simulink model "half_controlled_model"  (R2021b)
settings: Solver=VariableStepAuto  StartTime=0.0  StopTime=2  RelTol=1e-3
undefined symbols (not defined in the file): magnitude
libraries: spsCurrentMeasurementLib x2, spsDiodeLib x2, spsMeanLib x2, spsSeriesRLCBranchLib x2, spsThyristorLib x2, spsVoltageMeasurementLib x2, spsACVoltageSourceLib x1, spsDCMachineLib x1, spsDCVoltageSourceLib x1, spspowerguiLib x1
settings Model: Creator=ardak  LastModifiedBy=ardak

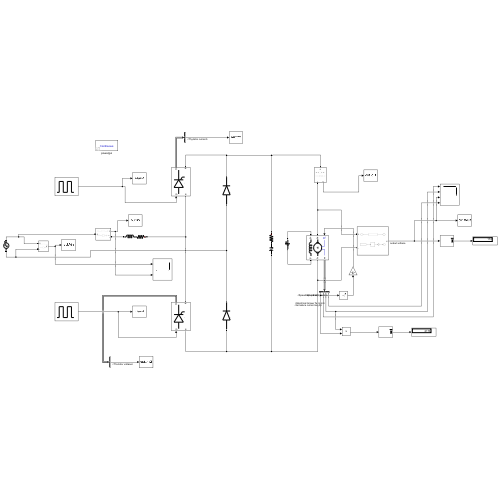
[thumbnail: Simulink's stored preview of the top-level diagram]
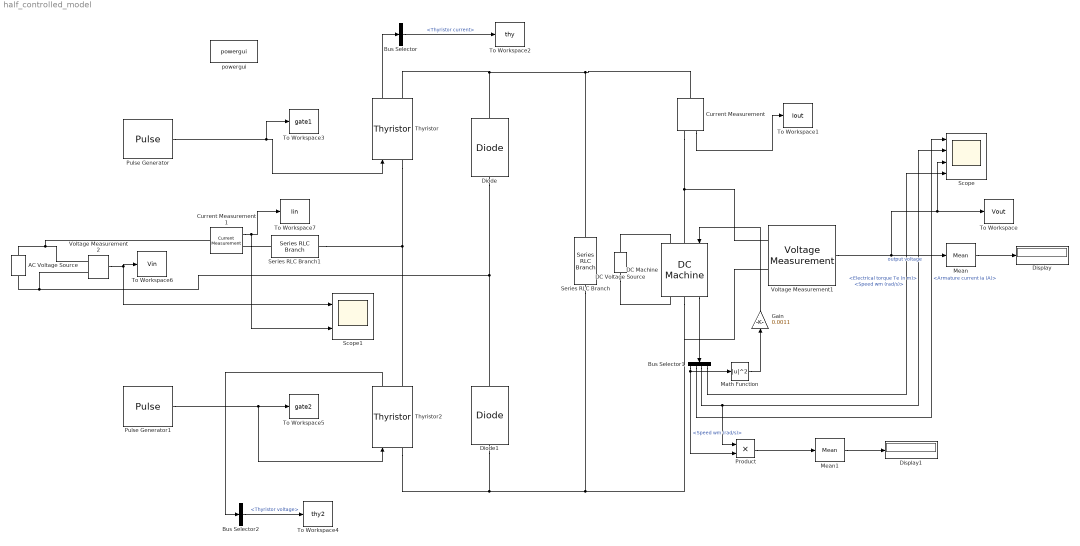
== system half_controlled_model ==
  AC Voltage Source : spsACVoltageSourceLib/AC Voltage Source  Amplitude=230*sqrt(2)  Phase=0  Frequency=50  SampleTime=1e-6  Measurements=None  BusType=swing  Pref=10e3  Qref=0  Qmin=-inf  Qmax=+inf
  Bus Selector : BusSelector  OutputSignals=Thyristor current
  Bus Selector1 : BusSelector  OutputSignals=Speed wm (rad/s),Armature current ia (A),Electrical torque Te (n m),Speed wm (rad/s)
  Bus Selector2 : BusSelector  OutputSignals=Thyristor voltage
  Current Measurement : spsCurrentMeasurementLib/Current Measurement  PhasorSimulation=off  OutputType=Complex  PSBequivalent=0
  Current Measurement1 : spsCurrentMeasurementLib/Current Measurement  PhasorSimulation=off  OutputType=Complex  PSBequivalent=0
  DC Machine : spsDCMachineLib/DC Machine  PresetModel=No  MechanicalLoad=Torque TL  FieldType=Wound  ShowDetailedParameters=on  MeasurementBus=off  RLa="[ 0.8  0.0125]"  RLf="[ 210  23]"  Laf=1.8  MachineConstant=Torque constant (N.m/A)  Ke=1.8  Kt=1.8  J=0.022  Bm=0.002953  Tf=0.5161  w0=1  Ifinit=0.714285714285714  TsPowergui=0  TsBlock=-1
  DC Voltage Source : spsDCVoltageSourceLib/DC Voltage Source  Amplitude=150  Measurements=None
  Diode : spsDiodeLib/Diode  Ron=0  Lon=0  Vf=1.2  IC=0  UseSnubber=0  Rs=inf  Cs=inf  Measurements=off
  Diode1 : spsDiodeLib/Diode  Ron=0  Lon=0  Vf=1.2  IC=0  UseSnubber=0  Rs=inf  Cs=inf  Measurements=off
  Display : Display
  Display1 : Display
  Gain : Gain  Gain=0.0011
  Math Function : Math  Operator=magnitude^2  SaturateOnIntegerOverflow=on
  Mean : spsMeanLib/Mean  Freq=60  Vinit=0  Ts=0
  Mean1 : spsMeanLib/Mean  Freq=60  Vinit=0  Ts=0
  Product : Product
  Pulse Generator : DiscretePulseGenerator  PulseType=Time based  Amplitude=200  Period=0.02  PulseWidth=20  PhaseDelay=0.0035
  Pulse Generator1 : DiscretePulseGenerator  PulseType=Time based  Amplitude=200  Period=0.02  PulseWidth=20  PhaseDelay=0.0135
  Scope : Scope  NumInputPorts=4
  Scope1 : Scope  NumInputPorts=2
  Series RLC Branch : spsSeriesRLCBranchLib/Series RLC Branch  LConnTagsString=__new0  RConnTagsString=__new0  BranchType=RC  Resistance=1  Inductance=1e-3  SetiL0=off  InitialCurrent=0  Capacitance=1360e-6  Setx0=off  InitialVoltage=0  Measurements=None
  Series RLC Branch1 : spsSeriesRLCBranchLib/Series RLC Branch  LConnTagsString=__new0  RConnTagsString=__new0  BranchType=RL  Resistance=1  Inductance=15e-3  SetiL0=off  InitialCurrent=0  Capacitance=1e-6  Setx0=off  InitialVoltage=0  Measurements=None
  Thyristor : spsThyristorLib/Thyristor  Ron=0.035  Lon=0  Vf=1.4  IC=0  Rs=inf  Cs=inf  Measurements=on
  Thyristor2 : spsThyristorLib/Thyristor  Ron=0.035  Lon=0  Vf=1.4  IC=0  Rs=inf  Cs=inf  Measurements=on
  To Workspace : ToWorkspace  VariableName=Vout  SampleTime=-1
      settings: Save2DSignal=2-D array (concatenate along first dimension)
  To Workspace1 : ToWorkspace  VariableName=Iout  SampleTime=-1
      settings: Save2DSignal=2-D array (concatenate along first dimension)
  To Workspace2 : ToWorkspace  VariableName=thy  SampleTime=-1
      settings: Save2DSignal=2-D array (concatenate along first dimension)
  To Workspace3 : ToWorkspace  VariableName=gate1  SampleTime=-1
      settings: Save2DSignal=2-D array (concatenate along first dimension)
  To Workspace4 : ToWorkspace  VariableName=thy2  SampleTime=-1
      settings: Save2DSignal=2-D array (concatenate along first dimension)
  To Workspace5 : ToWorkspace  VariableName=gate2  SampleTime=-1
      settings: Save2DSignal=2-D array (concatenate along first dimension)
  To Workspace6 : ToWorkspace  VariableName=Vin  SampleTime=-1
      settings: Save2DSignal=2-D array (concatenate along first dimension)
  To Workspace7 : ToWorkspace  VariableName=Iin  SampleTime=-1
      settings: Save2DSignal=2-D array (concatenate along first dimension)
  Voltage Measurement1 : spsVoltageMeasurementLib/Voltage Measurement  PhasorSimulation=off  OutputType=Complex  PSBequivalent=0
  Voltage Measurement2 : spsVoltageMeasurementLib/Voltage Measurement  PhasorSimulation=off  OutputType=Complex  PSBequivalent=0
  powergui : spspowerguiLib/powergui  Priority=1  SimulationMode=Continuous  SampleTime=5e-12  frequency=60  Iterations=50  frequencyindice=50  Pbase=100e6  ErrMax=1e-4  UnitsV=kV  UnitsW=MW  buscounter=0  FunctionMessages=off  echomessages=off  EnableUseOfTLC=off  CurrentSourceSwitches=off  DisableSnubberDevices=off  DisableRonSwitches=off  DisableVfSwitches=off  DisplayEquations=off  AutomaticDiscreteSolvers=off  SolverType=Tustin/Backward Euler (TBE)  Interpol=off  ExternalGateDelay=off  methode=off  Ts=100  x0status=blocks  SPID=on  SwTol=0  HookPort=off  NonlinearTolerance=1e-4  nMaxIteration=100  ContinueOnMaxIteration=off  RestoreLinks=warning  ResistiveCurrentMeasurement=off  Frange=[0:2:500]  Ylog=off  Xlog=on  ShowGrid=off  save=off  variable=ZData  structure=0  ZoomFFT=off  StartTime=0.0  cycles=1  DisplayStyle=1  fundamental=60  FreqAxis=off  MaxFrequency=1000  frequencyindicesteady=1  RmsSteady=1  display=off
  wires:
  Voltage Measurement1/1 -> Mean/1, To Workspace/1, Scope/3  "output voltage"
  Current Measurement/1 -> To Workspace1/1
  Pulse Generator/1 -> To Workspace3/1, Thyristor/1
  Pulse Generator1/1 -> To Workspace5/1, Thyristor2/1
  Mean/1 -> Display/1
  Thyristor/1 -> Bus Selector/1
  Thyristor2/1 -> Bus Selector2/1
  Bus Selector2/1 -> To Workspace4/1  "<Thyristor voltage>"
  Voltage Measurement2/1 -> Scope1/1, To Workspace6/1
  DC Machine/1 -> Bus Selector1/1
  Bus Selector1/1 -> Product/2, Math Function/1  "<Speed wm (rad/s)>"
  Math Function/1 -> Gain/1
  Gain/1 -> DC Machine/1
  Bus Selector1/4 -> Scope/4  "<Speed wm (rad/s)>"
  Bus Selector1/2 -> Scope/1  "<Armature current ia (A)>"
  Bus Selector1/3 -> Product/1, Scope/2  "<Electrical torque Te (n m)>"
  Mean1/1 -> Display1/1
  Product/1 -> Mean1/1
  Current Measurement1/1 -> Scope1/2, To Workspace7/1
  Bus Selector/1 -> To Workspace2/1  "<Thyristor current>"
  connections:
  Current Measurement/RConn1 -- DC Machine/LConn1 -- Voltage Measurement1/LConn1
  Thyristor2/LConn1 -- DC Machine/RConn1 -- Voltage Measurement1/LConn2 -- Series RLC Branch/RConn1 -- Diode1/LConn1
  Thyristor/LConn1 -- Thyristor2/RConn1 -- Series RLC Branch1/LConn1
  Diode/LConn1 -- AC Voltage Source/LConn1 -- Voltage Measurement2/LConn2 -- Diode1/RConn1
  DC Voltage Source/RConn1 -- DC Machine/LConn2
  DC Voltage Source/LConn1 -- DC Machine/RConn2
  Thyristor/RConn1 -- Series RLC Branch/LConn1 -- Current Measurement/LConn1 -- Diode/RConn1
  AC Voltage Source/RConn1 -- Current Measurement1/LConn1 -- Voltage Measurement2/LConn1
  Current Measurement1/RConn1 -- Series RLC Branch1/RConn1
